simulink model "soc_rfsoc_top"  (R2023b)
settings: Solver=VariableStepAuto  StartTime=0.0  StopTime=4e-3  RelTol=1e-3  EnableMultiTasking=on
PreLoadFcn:
  | FrameSize = 2048;
  | NumBuffers = 16;
  | downSamplingFactor = 64;
  | SrcSel = 0;
PostLoadFcn:
  | soc_rfsoc_init(bdroot);
InitFcn:
  | soc_rfsoc_init(bdroot);
model workspace (MAT data in the model file):
  mmap = soc.memmap.MemoryMap
  mmap.isMapValid = 1
  mmap.controllerInfo = soc.memmap.MemController
  mmap.controllerInfo.memPSRange = {'2', 'G'}
  mmap.controllerInfo.memPLBaseAddr = '0x500000000'
  mmap.controllerInfo.memPLRange = {'4', 'G'}
  mmap.controllerInfo.memPLBaseAddrMMU = {9, '0'}
  mmap.controllerInfo.regBaseAddr = '0xA0000000'
  mmap.controllerInfo.regAddrRange = {'256', 'M'}
  mmap.map(1) = soc.memmap.MapParams
  mmap.map(1).type = 'PS Memory Region'
  mmap.map(1).name = 'AXI4-Stream to Software'
  mmap.map(1).baseAddr = '0x00000000'
  mmap.map(1).range = {'128', 'K'}
  mmap.map(1).path = 'soc_rfsoc_top/AXI4-Stream to Software'
  mmap.map(2) = soc.memmap.MapParams
  mmap.map(2).type = 'PS Memory Region'
  mmap.map(2).name = 'Software to AXI4-Stream'
  mmap.map(2).baseAddr = '0x00020000'
  mmap.map(2).range = {'128', 'K'}
  mmap.map(2).path = 'soc_rfsoc_top/Software to AXI4-Stream'
  mmap.map(3) = soc.memmap.MapParams
  mmap.map(3).type = 'User Component'
  mmap.map(3).name = 'FPGA Tx-Rx Alg Wrapper'
  mmap.map(3).baseAddr = '0xA0000000'
  mmap.map(3).range = {'64', 'K'}
  mmap.map(3).path = 'soc_rfsoc_fpga/FPGA Tx-Rx Alg Wrapper'
  mmap.map(4) = soc.memmap.MapParams
  mmap.map(4).type = 'Implicit Component'
  mmap.map(4).name = 'AXI4-Stream to Software DMA S2MM'
  mmap.map(4).baseAddr = '0xA0010000'
  mmap.map(4).range = {'64', 'K'}
  mmap.map(5) = soc.memmap.MapParams
  mmap.map(5).type = 'Implicit Component'
  mmap.map(5).name = 'Software to AXI4-Stream DMA MM2S'
  mmap.map(5).baseAddr = '0xA0020000'
  mmap.map(5).range = {'64', 'K'}
  mmap.map(6) = soc.memmap.MapParams
  mmap.map(6).type = 'Implicit Component'
  mmap.map(6).name = 'RFDataConverter/s_axi'
  mmap.map(6).baseAddr = '0xA3C00000'
  mmap.map(6).range = {'256', 'K'}
  mwTaskManagerKernelLatency = 0
  socvcb = containers.Map
  socvcb.serialization.keys = {2.00024414062, 2.61853027344, 2.85791015625, 3.30261230469, 8.00073242188, 9.00073242188, 10.0029296875, 10.0031738281, 10.0078125, 11.0029296875, 11.0031738281, 11.0078125, 19.0009765625, 19.0014648438, 19.0017089844, 19.0018310547, 20.0009765625, 20.0012207031, 20.0013427734, 20.0015869141, 20.0017089844, 20.0043945312, 20.0052490234, 21.0001220703, 21.0004882812, 21.0007324219, 21.0008544922, 21.0009765625, 21.0010986328, 21.0013427734, 21.0014648438, 21.0017089844, 21.0018310547, 21.0025634766, 21.0028076172, 21.0040283203, 21.0043945312, 21.0045166016, 21.0052490234, 21.0067138672, 21.0076904297, 21.0122070312, 21.0130615234, 21.2208251953, 22.0001220703, 22.0004882812, 22.0006103516, 22.0008544922, 22.0009765625, 22.0013427734, 22.0017089844, 22.0018310547, 22.0024414062, 22.0025634766, 22.0028076172, 22.0040283203, 22.0045166016, 22.0052490234, 22.0067138672, 22.0076904297, 22.0122070312, 22.0130615234, 22.2208251953, 36.0002441406, 37.0003662109, 1663.81762695, 5736.00585938, 5737.00585938, 9227.89709473, 9749.0144043, 9749.01550293, 9750.0144043, 9750.01550293, 23272.0076904, 83164.0001221}
  socvcb.serialization.values : function handle (value not decoded)
  socvcb.serialization.uniformity = 0
  socvcb.serialization.keyType = 'double'
  socvcb.serialization.valueType = 'any'
undefined symbols (not defined in the file or in its folder): D1, Fs, I, m, n, P, Q
libraries: socmemlib x2, prociodatalib x2, proctasklib x1, xilinxrfsoclib x1, simulink x1
settings Model: Creator=The MathWorks, Inc.  LastModifiedBy=akroh
settings SolverCC: AlgebraicLoopSolver=TrustRegion  PositivePriorityOrder=on  AutoInsertRateTranBlk=on  MaxZcPerStep=1
settings DataIOCC: SaveFormat=StructureWithTime  ReturnWorkspaceOutputs=off
settings OptimizationCC: PassReuseOutputArgsAs=Individual arguments  MaxStackSize=64  EfficientTunableParamExpr=on
settings DebuggingCC: ParameterTunabilityLossMsg=error  UnconnectedInputMsg=warning  UnconnectedOutputMsg=warning  UnconnectedLineMsg=warning  ArithmeticOperatorsInVariantConditions=warning
settings HardwareCC: ProdBitPerLong=64  ProdLargestAtomicInteger=LongLong  ProdLargestAtomicFloat=Double  ProdLongLongMode=on  ProdHWDeviceType=ARM Compatible->ARM 64-bit (LP64)  HardwareBoardFeatureSet=SoCBlockset
settings ModelReferenceCC: EnableRefExpFcnMdlSchedulingChecks=on
settings SFSimCC: SimUseLocalCustomCode=off  CustomCodeUndefinedFunction=UseInterfaceOnly
settings RTWCC: Description=Embedded Coder  SystemTargetFile=ert.tlc  HardwareBoard=Xilinx Zynq UltraScale+ RFSoC ZCU111 Evaluation Kit  TLCOptions="-aInlineSetEventsForThisBaseRateFcn=TLC_FALSE -aSuppressMultiTaskScheduler=TLC_FALSE  -aRateBasedStepFcn=0"  TemplateMakefile=ert_default_tmf  GenerateReport=on  RTWUseLocalCustomCode=off  Toolchain=Linaro AArch64 Linux v6.3.1  IncludeHyperlinkInReport=on  LaunchReport=on  GenerateTraceInfo=on  GenerateTraceReport=on  GenerateTraceReportSl=on  GenerateTraceReportSf=on  GenerateTraceReportEml=on  DLArmComputeVersion=19.05
settings CodeAppCC: ForceParamTrailComments=on  IgnoreCustomStorageClasses=off  OperatorAnnotations=on  SimulinkDataObjDesc=on  SFDataObjDesc=on  InsertBlockDesc=on

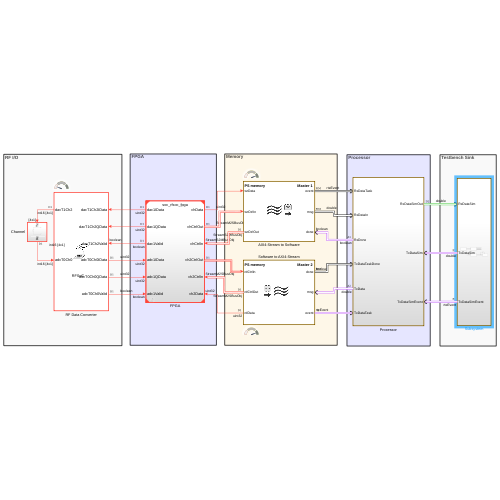
[thumbnail: Simulink's stored preview of the top-level diagram]
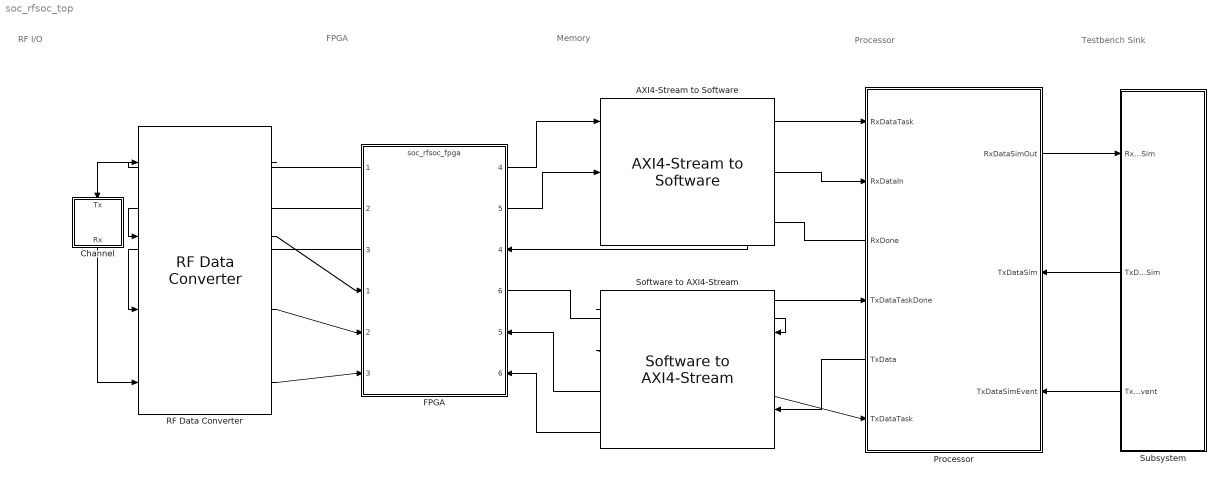
== system soc_rfsoc_top ==
  note: RF I/O
  note: Memory
  note: Processor
  note: FPGA
  note: Testbench Sink
  AXI4-Stream to Software : socmemlib/AXI4-Stream to Software  MemorySimulation=Burst accurate  MemorySelection=PS memory  MRNumBuffers=NumBuffers  BurstLengthWriterChIf=256  FIFODepthWriter=8  FIFOAFullDepthWriter=6  ICClockFrequencyWriter=100  ICDataWidthWriter=32  ChDimensionsWriterChIf=1  ChTypeWriterChIf=uint32  ChFrameSampleTimeWriterChIf=SampleTime  ChBitPackedWriterChIf=off  ChDimensionsReaderChIf=FrameSize  ChTypeReaderChIf=uint32  LastTargetBoard=Xilinx Zynq UltraScale+ RFSoC ZCU111 Evaluation Kit  MRRegionSize=131072  MRBufferSize=8192  DiagnosticLevel=No debug
  Channel : Subsystem
  FPGA : ModelReference  ModelNameDialog=soc_rfsoc_fpga.slx  SimulationMode=Normal  ModelReferenceVersion=7.14
      settings: PortSchema="{\"entries\":[{\"content\":{\"sides\":[{\"content\":{\"connectorIds\":[\"Out1\",\"Out2\",\"Out3\",\"In1\",\"In2\",\"In3\"]},\"type\":\"ConnectorPlacement.EquallySpacedRectSide\",\"uuid\":\"5cb1a72a-01db-451a-a1d5-13c90475b746\"},{\"content\":{\"connectorIds\":[\"Out4\",\"Out5\",\"In4\",\"Out6\",\"In5\",\"In6\"],\"side\":\"RIGHT\"},\"type\":\"ConnectorPlacement.EquallySpacedRectSide\",\"uuid\":\"0cc5c425-085f-4d55-8809-74a02be1a373\"},{\"content\":{\"side\":\"TOP\"},\"type\":\"ConnectorPlacement.EquallySpacedRectSide\",\"uuid\":\"74405138-49c7-488d-8705-1658c6d2c17e\"},{\"content\":{\"side\":\"BOTTOM\"},\"type\":\"ConnectorPlacement.EquallySpacedRectSide\",\"uuid\":\"41d3b708-b00f-42a5-bfad-1616ef33dc5f\"}]},\"type\":\"ConnectorPlacement.EquallySpacedConnector\",\"uuid\":\"fa285e06-79f7-4ad6-b6b8-2363bd8486be\"}],\"packageUris\":[\"http://schema.mathworks.com/mf0/Connector/R2020b\"],\"version\":\"1.0\"}"
  Processor : Subsystem
      settings: PortSchema="{\"entries\":[{\"content\":{\"sides\":[{\"content\":{\"connectorIds\":[\"In1\",\"In2\",\"Out2\",\"In3\",\"Out3\",\"In4\"]},\"type\":\"ConnectorPlacement.EquallySpacedRectSide\",\"uuid\":\"c6517cf8-029b-42a5-8e0a-4a74babda661\"},{\"content\":{\"connectorIds\":[\"Out1\",\"In5\",\"In6\"],\"side\":\"RIGHT\"},\"type\":\"ConnectorPlacement.EquallySpacedRectSide\",\"uuid\":\"16c669d3-b531-49c5-97c0-aad9de53fc76\"},{\"content\":{\"side\":\"TOP\"},\"type\":\"ConnectorPlacement.EquallySpacedRectSide\",\"uuid\":\"ee928f87-c942-476b-86c6-8f97cdee9f2e\"},{\"content\":{\"side\":\"BOTTOM\"},\"type\":\"ConnectorPlacement.EquallySpacedRectSide\",\"uuid\":\"ef0c39df-7d54-4afb-ba81-784fc61f5805\"}]},\"type\":\"ConnectorPlacement.EquallySpacedConnector\",\"uuid\":\"c956b2ab-b210-4cbd-a6ac-ba45bfad9e74\"}],\"packageUris\":[\"http://schema.mathworks.com/mf0/Connector/R2020b\"],\"version\":\"1.0\"}"
  RF Data Converter : xilinxrfsoclib/RF Data Converter  RFDCSim=Pass-through  tabPromptsCB=0  RFInterface=Customize  digitalInterface=I/Q  dac11Enable=off  dac12Enable=off  dac13Enable=off  dac14Enable=off  dac21Enable=off  dac22Enable=off  dac23Enable=on  dac24Enable=off  dac31Enable=off  dac32Enable=off  dac33Enable=off  dac34Enable=off  dac41Enable=off  dac42Enable=off  dac43Enable=off  dac44Enable=off  matchDACParam=on  dacSampleRate=1024  interpolationMode=4  dacSamplesPerCycle=2  dacMixerType=Coarse  dacMixerMode=I/Q->Real  dacMixerFrequency=Fs/4  dacNCOFrequency=0  dacNCOPhase=0  invertSyncFilter=off  dacTile1SampleRate=1000  dac11InterpolationMode=2  dac11SamplesPerCycle=2  dac11MixerType=Coarse  dac11MixerMode=I/Q->Real  dac11MixerFrequency=Fs/2  dac11NCOFrequency=0  dac11NCOPhase=0  dac11InvertSyncFilter=off  dac12InterpolationMode=2  dac12SamplesPerCycle=2  dac12MixerType=Coarse  dac12MixerMode=I/Q->Real  dac12MixerFrequency=Fs/2  dac12NCOFrequency=0  dac12NCOPhase=0  dac12InvertSyncFilter=off  dac13InterpolationMode=2  dac13SamplesPerCycle=2  dac13MixerType=Coarse  dac13MixerMode=I/Q->Real  dac13MixerFrequency=Fs/2  dac13NCOFrequency=0  dac13NCOPhase=0  dac13InvertSyncFilter=off  dac14InterpolationMode=2  dac14SamplesPerCycle=2  dac14MixerType=Coarse  dac14MixerMode=I/Q->Real  dac14MixerFrequency=Fs/2  dac14NCOFrequency=0  dac14NCOPhase=0  dac14InvertSyncFilter=off  dacTile2SampleRate=1000  dac21InterpolationMode=2  dac21SamplesPerCycle=2  dac21MixerType=Coarse  dac21MixerMode=I/Q->Real  dac21MixerFrequency=Fs/2  dac21NCOFrequency=0  dac21NCOPhase=0  dac21InvertSyncFilter=off  dac22InterpolationMode=2  dac22SamplesPerCycle=2  dac22MixerType=Coarse  dac22MixerMode=I/Q->Real  dac22MixerFrequency=Fs/2  dac22NCOFrequency=0  dac22NCOPhase=0  dac22InvertSyncFilter=off  dac23InterpolationMode=2  dac23SamplesPerCycle=2  dac23MixerType=Coarse  dac23MixerMode=I/Q->Real  dac23MixerFrequency=Fs/2  dac23NCOFrequency=0  dac23NCOPhase=0  dac23InvertSyncFilter=off  dac24InterpolationMode=2  dac24SamplesPerCycle=2  dac24MixerType=Coarse  dac24MixerMode=I/Q->Real  dac24MixerFrequency=Fs/2  dac24NCOFrequency=0  dac24NCOPhase=0  dac24InvertSyncFilter=off  dacTile3SampleRate=1000  dac31InterpolationMode=2  dac31SamplesPerCycle=2  dac31MixerType=Coarse  dac31MixerMode=I/Q->Real  dac31MixerFrequency=Fs/2  dac31NCOFrequency=0  dac31NCOPhase=0  dac31InvertSyncFilter=off  dac32InterpolationMode=2  dac32SamplesPerCycle=2  dac32MixerType=Coarse  dac32MixerMode=I/Q->Real  dac32MixerFrequency=Fs/2  dac32NCOFrequency=0  dac32NCOPhase=0  dac32InvertSyncFilter=off  dac33InterpolationMode=2  dac33SamplesPerCycle=2  dac33MixerType=Coarse  dac33MixerMode=I/Q->Real  dac33MixerFrequency=Fs/2  dac33NCOFrequency=0  dac33NCOPhase=0  dac33InvertSyncFilter=off  dac34InterpolationMode=2  dac34SamplesPerCycle=2  dac34MixerType=Coarse  dac34MixerMode=I/Q->Real  dac34MixerFrequency=Fs/2  dac34NCOFrequency=0  dac34NCOPhase=0  dac34InvertSyncFilter=off  dacTile4SampleRate=1000  dac41InterpolationMode=2  dac41SamplesPerCycle=2  dac41MixerType=Coarse  dac41MixerMode=I/Q->Real  dac41MixerFrequency=Fs/2  dac41NCOFrequency=0  dac41NCOPhase=0  dac41InvertSyncFilter=off  dac42InterpolationMode=2  dac42SamplesPerCycle=2  dac42MixerType=Coarse  dac42MixerMode=I/Q->Real  dac42MixerFrequency=Fs/2  dac42NCOFrequency=0  dac42NCOPhase=0  dac42InvertSyncFilter=off  dac43InterpolationMode=2  dac43SamplesPerCycle=2  dac43MixerType=Coarse  dac43MixerMode=I/Q->Real  dac43MixerFrequency=Fs/2  dac43NCOFrequency=0  dac43NCOPhase=0  dac43InvertSyncFilter=off  dac44InterpolationMode=2  dac44SamplesPerCycle=2  dac44MixerType=Coarse  dac44MixerMode=I/Q->Real  dac44MixerFrequency=Fs/2  dac44NCOFrequency=0  dac44NCOPhase=0  dac44InvertSyncFilter=off  adc11Enable=on  adc12Enable=off  adc13Enable=off  adc14Enable=off  adc21Enable=off  adc22Enable=off  adc23Enable=off  adc24Enable=off  adc31Enable=off  adc32Enable=off  adc33Enable=off  adc34Enable=off  adc41Enable=off  adc42Enable=off  adc43Enable=off  adc44Enable=off  adcOutUnpackedData=off  matchADCParam=on  adcSampleRate=1024  decimationMode=4  adcSamplesPerCycle=2  adcMixerType=Coarse  adcMixerMode=Real->I/Q  adcMixerFrequency=-Fs/4  adcNCOFrequency=0  adcNCOPhase=0  adcTile1SampleRate=1000  adc11DecimationMode=2  adc11SamplesPerCycle=2  adc11MixerType=Coarse  adc11MixerMode=Real->I/Q  adc11MixerFrequency=Fs/2  adc11NCOFrequency=0  adc11NCOPhase=0  adc12DecimationMode=2  adc12SamplesPerCycle=2  adc12MixerType=Coarse  adc12MixerMode=Real->I/Q  adc12MixerFrequency=Fs/2  adc12NCOFrequency=0  adc12NCOPhase=0  adc13DecimationMode=2  adc13SamplesPerCycle=2  adc13MixerType=Coarse  adc13MixerMode=Real->I/Q  adc13MixerFrequency=Fs/2  adc13NCOFrequency=0  adc13NCOPhase=0  adc14DecimationMode=2  adc14SamplesPerCycle=2  adc14MixerType=Coarse  adc14MixerMode=Real->I/Q  adc14MixerFrequency=Fs/2  adc14NCOFrequency=0  adc14NCOPhase=0  adcTile2SampleRate=1000  adc21DecimationMode=2  adc21SamplesPerCycle=2  adc21MixerType=Coarse  adc21MixerMode=Real->I/Q  adc21MixerFrequency=Fs/2  adc21NCOFrequency=0  adc21NCOPhase=0  adc22DecimationMode=2  adc22SamplesPerCycle=2  adc22MixerType=Coarse  adc22MixerMode=Real->I/Q  adc22MixerFrequency=Fs/2  adc22NCOFrequency=0  adc22NCOPhase=0  adc23DecimationMode=2  adc23SamplesPerCycle=2  adc23MixerType=Coarse  adc23MixerMode=Real->I/Q  adc23MixerFrequency=Fs/2  adc23NCOFrequency=0  adc23NCOPhase=0  adc24DecimationMode=2  adc24SamplesPerCycle=2  adc24MixerType=Coarse  adc24MixerMode=Real->I/Q  adc24MixerFrequency=Fs/2  adc24NCOFrequency=0  adc24NCOPhase=0  adcTile3SampleRate=1000  adc31DecimationMode=2  adc31SamplesPerCycle=2  adc31MixerType=Coarse  adc31MixerMode=Real->I/Q  adc31MixerFrequency=Fs/2  adc31NCOFrequency=0  adc31NCOPhase=0  adc32DecimationMode=2  adc32SamplesPerCycle=2  adc32MixerType=Coarse  adc32MixerMode=Real->I/Q  adc32MixerFrequency=Fs/2  adc32NCOFrequency=0  adc32NCOPhase=0  adc33DecimationMode=2  adc33SamplesPerCycle=2  adc33MixerType=Coarse  adc33MixerMode=Real->I/Q  adc33MixerFrequency=Fs/2  adc33NCOFrequency=0  adc33NCOPhase=0  adc34DecimationMode=2  adc34SamplesPerCycle=2  adc34MixerType=Coarse  adc34MixerMode=Real->I/Q  adc34MixerFrequency=Fs/2  adc34NCOFrequency=0  adc34NCOPhase=0  adcTile4SampleRate=1000  adc41DecimationMode=2  adc41SamplesPerCycle=2  adc41MixerType=Coarse  adc41MixerMode=Real->I/Q  adc41MixerFrequency=Fs/2  adc41NCOFrequency=0  adc41NCOPhase=0  adc42DecimationMode=2  adc42SamplesPerCycle=2  adc42MixerType=Coarse  adc42MixerMode=Real->I/Q  adc42MixerFrequency=Fs/2  adc42NCOFrequency=0  adc42NCOPhase=0  adc43DecimationMode=2  adc43SamplesPerCycle=2  adc43MixerType=Coarse  adc43MixerMode=Real->I/Q  adc43MixerFrequency=Fs/2  adc43NCOFrequency=0  adc43NCOPhase=0  adc44DecimationMode=2  adc44SamplesPerCycle=2  adc44MixerType=Coarse  adc44MixerMode=Real->I/Q  adc44MixerFrequency=Fs/2  adc44NCOFrequency=0  adc44NCOPhase=0  multiTileSync=off  externalPLL=off  dacRealTimeNCOPortsEnable=off  adcRealTimeNCOPortsEnable=off  adcRealTimePortsEnable=off  adcThresholdMode=Sticky over  adcThreshold1=0  adcDelayCounter=0  adcThreshold2Mode=Sticky over  adcThreshold2=0  adcThreshold2DelayCounter=0  adc11ThresholdMode=Sticky over  adc11Threshold1=0  adc11DelayCounter=0  adc11Threshold2Mode=Sticky over  adc11Threshold2=0  adc11Threshold2DelayCounter=0  adc12ThresholdMode=Sticky over  adc12Threshold1=0  adc12DelayCounter=0  adc12Threshold2Mode=Sticky over  adc12Threshold2=0  adc12Threshold2DelayCounter=0  adc13ThresholdMode=Sticky over  adc13Threshold1=0  adc13DelayCounter=0  adc13Threshold2Mode=Sticky over  adc13Threshold2=0  adc13Threshold2DelayCounter=0  adc14ThresholdMode=Sticky over  adc14Threshold1=0  adc14DelayCounter=0  adc14Threshold2Mode=Sticky over  adc14Threshold2=0  adc14Threshold2DelayCounter=0  adc21ThresholdMode=Sticky over  adc21Threshold1=0  adc21DelayCounter=0  adc21Threshold2Mode=Sticky over  adc21Threshold2=0  adc21Threshold2DelayCounter=0  adc22ThresholdMode=Sticky over  adc22Threshold1=0  adc22DelayCounter=0  adc22Threshold2Mode=Sticky over  adc22Threshold2=0  adc22Threshold2DelayCounter=0  adc23ThresholdMode=Sticky over  adc23Threshold1=0  adc23DelayCounter=0  adc23Threshold2Mode=Sticky over  adc23Threshold2=0  adc23Threshold2DelayCounter=0  adc24ThresholdMode=Sticky over  adc24Threshold1=0  adc24DelayCounter=0  adc24Threshold2Mode=Sticky over  adc24Threshold2=0  adc24Threshold2DelayCounter=0  adc31ThresholdMode=Sticky over  adc31Threshold1=0  adc31DelayCounter=0  adc31Threshold2Mode=Sticky over  adc31Threshold2=0  adc31Threshold2DelayCounter=0  adc32ThresholdMode=Sticky over  adc32Threshold1=0  adc32DelayCounter=0  adc32Threshold2Mode=Sticky over  adc32Threshold2=0  adc32Threshold2DelayCounter=0  adc33ThresholdMode=Sticky over  adc33Threshold1=0  adc33DelayCounter=0  adc33Threshold2Mode=Sticky over  adc33Threshold2=0  adc33Threshold2DelayCounter=0  adc34ThresholdMode=Sticky over  adc34Threshold1=0  adc34DelayCounter=0  adc34Threshold2Mode=Sticky over  adc34Threshold2=0  adc34Threshold2DelayCounter=0  adc41ThresholdMode=Sticky over  adc41Threshold1=0  adc41DelayCounter=0  adc41Threshold2Mode=Sticky over  adc41Threshold2=0  adc41Threshold2DelayCounter=0  adc42ThresholdMode=Sticky over  adc42Threshold1=0  adc42DelayCounter=0  adc42Threshold2Mode=Sticky over  adc42Threshold2=0  adc42Threshold2DelayCounter=0  adc43ThresholdMode=Sticky over  adc43Threshold1=0  adc43DelayCounter=0  adc43Threshold2Mode=Sticky over  adc43Threshold2=0  adc43Threshold2DelayCounter=0  adc44ThresholdMode=Sticky over  adc44Threshold1=0  adc44DelayCounter=0  adc44Threshold2Mode=Sticky over  adc44Threshold2=0  adc44Threshold2DelayCounter=0
  Software to AXI4-Stream : socmemlib/Software to AXI4-Stream  MemorySimulation=Burst accurate  MemorySelection=PS memory  MRNumBuffers=NumBuffers  BurstLengthReaderChIf=256  FIFODepthReader=8  FIFOAFullDepthReader=6  ICClockFrequencyReader=100  ICDataWidthReader=32  ChDimensionsWriterChIf=FrameSize  ChTypeWriterChIf=uint32  ChDimensionsReaderChIf=1  ChTypeReaderChIf=uint32  ChFrameSampleTimeReaderChIf=SampleTime  ChBitPackedReaderChIf=off  LastTargetBoard=Xilinx Zynq UltraScale+ RFSoC ZCU111 Evaluation Kit  MRRegionSize=131072  MRBufferSize=8192  DiagnosticLevel=No debug
  Subsystem : Subsystem
      settings: PortSchema="{\"entries\":[{\"content\":{\"sides\":[{\"content\":{\"connectorIds\":[\"In1\",\"Out1\",\"Out2\"]},\"type\":\"ConnectorPlacement.EquallySpacedRectSide\",\"uuid\":\"792ba10f-334c-4272-ab3e-edc99960d88d\"},{\"content\":{\"side\":\"RIGHT\"},\"type\":\"ConnectorPlacement.EquallySpacedRectSide\",\"uuid\":\"7e309716-18be-4699-ada9-d1cfe272fe72\"},{\"content\":{\"side\":\"TOP\"},\"type\":\"ConnectorPlacement.EquallySpacedRectSide\",\"uuid\":\"a79eced7-7557-4ca7-b528-e21b47b4bb96\"}]},\"type\":\"ConnectorPlacement.EquallySpacedConnector\",\"uuid\":\"f3eafb69-b6be-42bf-bcff-a3984c3a0506\"}],\"packageUris\":[\"http://schema.mathworks.com/mf0/Connector/R2020b\"],\"version\":\"1.0\"}"
  wires:
  RF Data Converter/1 -> Channel/1(Tx)
  Processor/1(RxDataSimOut) -> Subsystem/1(RxDataSim)
  FPGA/4 -> AXI4-Stream to Software/1
  FPGA/5 -> AXI4-Stream to Software/2
  AXI4-Stream to Software/1 -> Processor/1(RxDataTask)
  AXI4-Stream to Software/2 -> Processor/2(RxDataIn)
  Processor/2(RxDone) -> AXI4-Stream to Software/3
  RF Data Converter/2 -> FPGA/1
  Channel/1(Rx) -> RF Data Converter/4
  RF Data Converter/3 -> FPGA/2
  RF Data Converter/4 -> FPGA/3
  AXI4-Stream to Software/3 -> FPGA/4
  FPGA/1 -> RF Data Converter/1
  FPGA/2 -> RF Data Converter/2
  FPGA/3 -> RF Data Converter/3
  Software to AXI4-Stream/1 -> FPGA/6
  Software to AXI4-Stream/2 -> FPGA/5
  FPGA/6 -> Software to AXI4-Stream/2
  Software to AXI4-Stream/3 -> Processor/4(TxDataTask)
  Software to AXI4-Stream/4 -> Processor/3(TxDataTaskDone)
  Processor/3(TxData) -> Software to AXI4-Stream/1
  Subsystem/1(TxDataSim) -> Processor/5(TxDataSim)
  Subsystem/2(TxDataSimEvent) -> Processor/6(TxDataSimEvent)

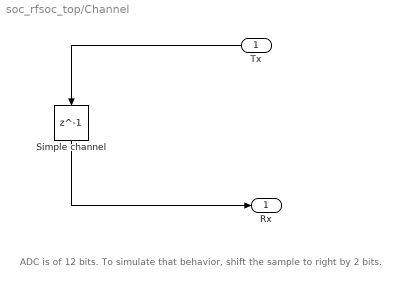
== system soc_rfsoc_top/Channel ==
  note: ADC is of 12 bits. To simulate that behavior, shift the sample to right by 2 bits.
  Tx : Inport
  Simple channel : Delay  DelayLength=1
  Rx : Outport  VectorParamsAs1DForOutWhenUnconnected=off
  wires:
  Tx/1 -> Simple channel/1
  Simple channel/1 -> Rx/1

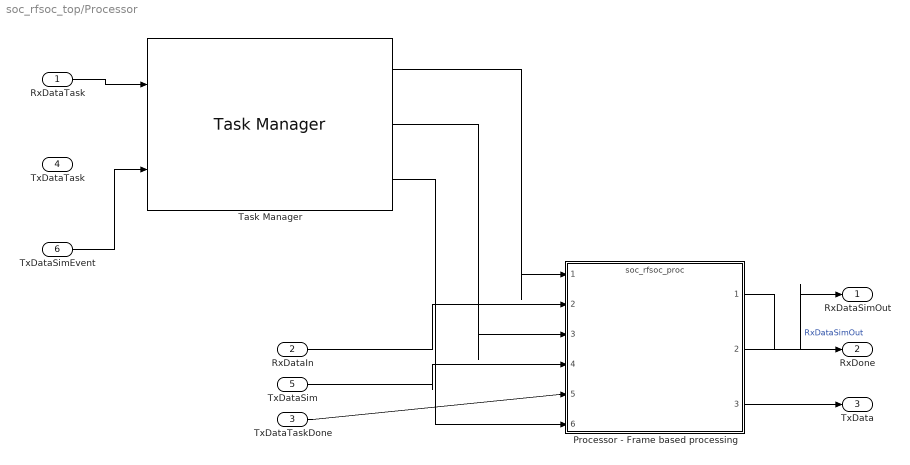
== system soc_rfsoc_top/Processor ==
  RxDataTask : Inport
  RxDataIn : Inport  Port=2
  TxDataTaskDone : Inport  Port=3
  TxDataTask : Inport  Port=4
  TxDataSim : Inport  Port=5
  TxDataSimEvent : Inport  Port=6
  Processor - Frame based processing : ModelReference  InputPortMessageModes=n,m,n,m,m,n  OutputPortMessageModes=m,m,m  ModelNameDialog=soc_rfsoc_proc.slx  SimulationMode=Normal  ScheduleRates=on  CachedPortDiscreteRates=[0.001]  ModelEventPortInfo=P:D1[0.001][0][0]  ModelReferenceVersion=7.38
  Task Manager : proctasklib/Task Manager  AllTaskData="[{\"taskName\":\"DataReadTask\",\"taskType\":\"Event-driven\",\"taskEvent\":\"DataReadTaskEvent\",\"taskPeriod\":\"0.1\",\"taskPriority\":\"50\",\"coreSelection\":\"Specified core\",\"coreNum\":\"0\",\"dropOverranTasks\":false,\"playbackRecorded\":false,\"diagnosticsFile\":\"\",\"taskDurationSource\":\"Dialog\",\"taskDuration\":0.000101031,\"taskDurationDeviation\":1.3727E-5,\"logExecutionData\":true,\"logDroppedTasks\":false,\"version\":\"2.6\",\"taskDurationData\":{\"percent\":[\"100\"],\"mean\":[\"0.5e-3\"],\"dev\":[\"0\"],\"min\":[\"0.5e-3\"],\"max\":[\"0.5e-3\"]},\"taskEventSource\":\"AXI4-Stream to Software\",\"taskEventSourceAssignmentType\":\"AutoAssigned\",\"taskEventSourceType\":\"Stream\",\"taskEventGroup\":\"Unspecified\",\"taskEventInterrupt\":\"Unspecified\",\"taskEventOrder\":1,\"taskDisablePremption\":false,\"taskClearInterruptFlagsAtEndOfEvent\":false},{\"taskName\":\"DataWriteTask\",\"taskType\":\"Event-driven\",\"taskEvent\":\"DataWriteTaskEvent\",\"taskPeriod\":\"0.1\",\"taskPriority\":\"52\",\"coreSelection\":\"Specified core\",\"coreNum\":\"0\",\"dropOverranTasks\":false,\"playbackRecorded\":false,\"diagnosticsFile\":\"\",\"taskDurationSource\":\"Dialog\",\"taskDuration\":1E-6,\"taskDurationDeviation\":0,\"logExecutionData\":true,\"logDroppedTasks\":false,\"version\":\"2.6\",\"taskDurationData\":{\"percent\":\"100\",\"mean\":\"1e-06\",\"dev\":\"0\",\"min\":\"1e-06\",\"max\":\"1e-06\"},\"taskEventSource\":\"IO Data Source\",\"taskEventSourceAssignmentType\":\"AutoAssigned\",\"taskEventSourceType\":\"TCP\",\"taskEventGroup\":\"Unspecified\",\"taskEventInterrupt\":\"Unspecified\",\"taskEventOrder\":1,\"taskDisablePremption\":false,\"taskClearInterruptFlagsAtEndOfEvent\":false},{\"taskName\":\"Periodic\",\"taskType\":\"Timer-driven\",\"taskEvent\":\"PeriodicEvent\",\"taskPeriod\":\"1e-3\",\"taskPriority\":\"53\",\"coreSelection\":\"Specified core\",\"coreNum\":\"0\",\"dropOverranTasks\":false,\"playbackRecorded\":false,\"diagnosticsFile\":\"\",\"taskDurationSource\":\"Dialog\",\"taskDuration\":1E-6,\"taskDurationDeviation\":0,\"logExecutionData\":true,\"logDroppedTasks\":false,\"version\":\"2.6\",\"taskDurationData\":{\"percent\":\"100\",\"mean\":\"1e-06\",\"dev\":\"0\",\"min\":\"1e-06\",\"max\":\"1e-06\"},\"taskEventSource\":\"Internal\",\"taskEventSourceAssignmentType\":\"AutoAssigned\",\"taskEventSourceType\":\"Unspecified\",\"taskEventGroup\":\"Unspecified\",\"taskEventInterrupt\":\"Unspecified\",\"taskEventOrder\":1,\"taskDisablePremption\":false,\"taskClearInterruptFlagsAtEndOfEvent\":false}]"  EnableTaskSimulation=on  StreamToSDI=on  WriteToFile=off  OverwriteFile=off  SupportEventPorts=on  UseScheduleEditor=off  CustomizationInfo=''
  RxDataSimOut : Outport  VectorParamsAs1DForOutWhenUnconnected=off
  RxDone : Outport  Port=2  VectorParamsAs1DForOutWhenUnconnected=off
  TxData : Outport  Port=3
  wires:
  RxDataIn/1 -> Processor - Frame based processing/2
  RxDataTask/1 -> Task Manager/1
  Task Manager/1 -> Processor - Frame based processing/1
  Processor - Frame based processing/1 -> RxDone/1
  Processor - Frame based processing/2 -> RxDataSimOut/1  "RxDataSimOut"
  Task Manager/2 -> Processor - Frame based processing/3
  Processor - Frame based processing/3 -> TxData/1
  TxDataSim/1 -> Processor - Frame based processing/4
  TxDataTaskDone/1 -> Processor - Frame based processing/5
  TxDataSimEvent/1 -> Task Manager/2
  Task Manager/3 -> Processor - Frame based processing/6

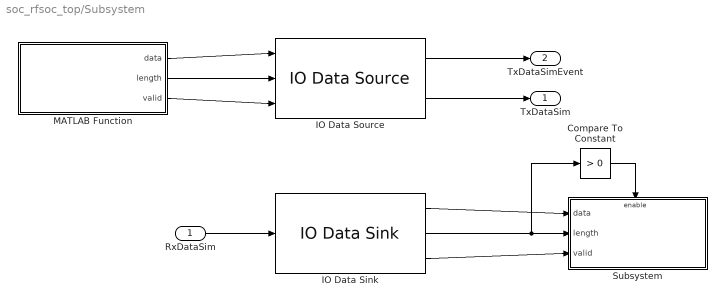
== system soc_rfsoc_top/Subsystem ==
  RxDataSim : Inport
  Compare To Constant : simulink/Logic and Bit Operations/Compare To Constant  relop=>  const=0  OutDataTypeStr=boolean
  IO Data Sink : prociodatalib/IO Data Sink  OutputSink=To output port  DataTypeStr=uint32  Dimensions=FrameSize  DeviceType=TCP  EventDataPort=Data  QueueLength=8  SampleTime=-1  EnableDonePort=off
  IO Data Source : prociodatalib/IO Data Source  InputSource=From input port  Value=uint32(1:1024)  ObjectName=[]  DeviceType=TCP  ShowEventPort=off  EventDataPort=Data and Event  QueueLength=8  DataTypeStr=uint32  Dimensions=1024  ShowDonePort=off  SampleTime=-1  InternalSampleTime=-1
  MATLAB Function : MATLAB Function  TreatAsAtomicUnit=on  SystemSampleTime=1e-3
  Subsystem : Subsystem
  TxDataSim : Outport
  TxDataSimEvent : Outport  Port=2
  wires:
  RxDataSim/1 -> IO Data Sink/1
  IO Data Source/2 -> TxDataSim/1
  MATLAB Function/1(data) -> IO Data Source/1
  MATLAB Function/2(length) -> IO Data Source/2
  MATLAB Function/3(valid) -> IO Data Source/3
  IO Data Source/1 -> TxDataSimEvent/1
  IO Data Sink/1 -> Subsystem/1(data)
  IO Data Sink/2 -> Compare To Constant/1, Subsystem/2(length)
  IO Data Sink/3 -> Subsystem/3(valid)
  Compare To Constant/1 -> Subsystem/Enable

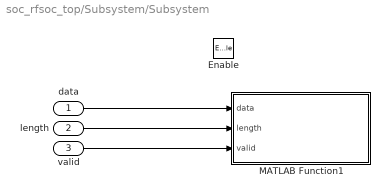
== system soc_rfsoc_top/Subsystem/Subsystem ==
  data : Inport
  length : Inport  Port=2
  valid : Inport  Port=3
  Enable : EnablePort
  MATLAB Function1 : MATLAB Function  TreatAsAtomicUnit=on
  wires:
  data/1 -> MATLAB Function1/1(data)
  length/1 -> MATLAB Function1/2(length)
  valid/1 -> MATLAB Function1/3(valid)

== matlab function soc_rfsoc_top/Subsystem/MATLAB Function ==
  data: data output; length output; valid output
function [data, length, valid] = fcn()

persistent iteration;

if isempty(iteration)
    iteration = uint32(1);
end


length = 2048;
data = uint32((1:length))  + iteration;
valid = 1;
disp(sprintf("TCP frame sent (#%u; %u)", iteration, data(1)))
%disp(data)

iteration = iteration + 1;

== matlab function soc_rfsoc_top/Subsystem/Subsystem/MATLAB Function1 ==
  data: data input; length input; valid input
function fcn(data, length, valid)
disp("Frame received");
disp(data);
%disp(length);
%disp(valid);
